simulink model "tutorial2"  (R2015a)
settings: Solver=ode45  StartTime=0.0  StopTime=24  RelTol=1e-3
model workspace (MAT data in the model file):
  T_heater = 50
  M_heater_air = 3600
  c_air = 1005.4
  m_room_air = 1470
  T_roomIC = 20
  R_equivalent = 4.329e-07
settings Model: Creator=eric  LastModifiedBy=eric

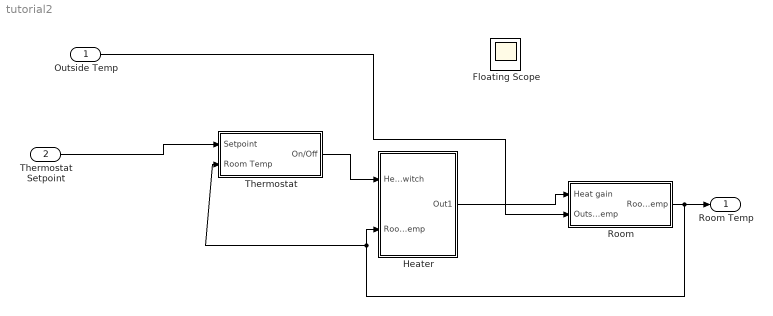
== system tutorial2 ==
  Outside Temp : Inport
  Thermostat Setpoint : Inport  Port=2
  Floating Scope : Scope  NumInputPorts=2
      settings: Floating=on  YMin=0~0  YMax=50~100000000
  Heater : Subsystem
  Room : Subsystem
  Thermostat : Subsystem
  Room Temp : Outport
  wires:
  Heater/1(Out1) -> Room/1(Heat gain)
  Thermostat/1(On/Off) -> Heater/1(Heater Switch)
  Room/1(Room Temp) -> Room Temp/1, Thermostat/2(Room Temp), Heater/2(Room Temp)
  Outside Temp/1 -> Room/2(Outside Temp)
  Thermostat Setpoint/1 -> Thermostat/1(Setpoint)

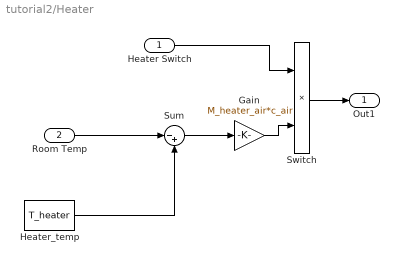
== system tutorial2/Heater ==
  Heater Switch : Inport
  Room Temp : Inport  Port=2
  Gain : Gain  Gain=M_heater_air*c_air
  Heater_temp : Constant  Value=T_heater
  Sum : Sum  Inputs=|-+
  Switch : Product
  Out1 : Outport
  wires:
  Heater Switch/1 -> Switch/1
  Room Temp/1 -> Sum/1
  Heater_temp/1 -> Sum/2
  Sum/1 -> Gain/1
  Gain/1 -> Switch/2
  Switch/1 -> Out1/1

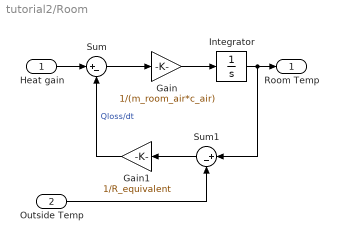
== system tutorial2/Room ==
  Heat gain : Inport
  Outside Temp : Inport  Port=2
  Gain : Gain  Gain=1/(m_room_air*c_air)
  Gain1 : Gain  Gain=1/R_equivalent
  Integrator : Integrator  InitialCondition=20
  Sum : Sum  Inputs=|+-
  Sum1 : Sum  Inputs=|+-
  Room Temp : Outport
  wires:
  Heat gain/1 -> Sum/1
  Sum/1 -> Gain/1
  Gain/1 -> Integrator/1
  Integrator/1 -> Sum1/1, Room Temp/1
  Gain1/1 -> Sum/2  "Qloss/dt"
  Sum1/1 -> Gain1/1
  Outside Temp/1 -> Sum1/2

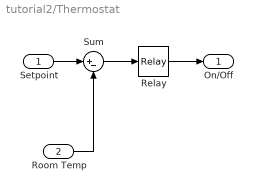
== system tutorial2/Thermostat ==
  Setpoint : Inport
  Room Temp : Inport  Port=2
  Relay : Relay  OnSwitchValue=2  OffSwitchValue=-2
  Sum : Sum  Inputs=|+-
  On/Off : Outport
  wires:
  Setpoint/1 -> Sum/1
  Room Temp/1 -> Sum/2
  Sum/1 -> Relay/1
  Relay/1 -> On/Off/1
